simulink model "OkidniStepen"  (R2014b)
settings: Solver=ode5  StartTime=0.0  StopTime=0.1  FixedStep=10e-6  RelTol=1e-3
values from neighbouring files (symbols this model uses):
  f = 50    [Parametri.m]
  Vmax = 220*sqrt(2)    [Parametri.m]
settings Model: Creator=Zorana  LastModifiedBy=Zorana

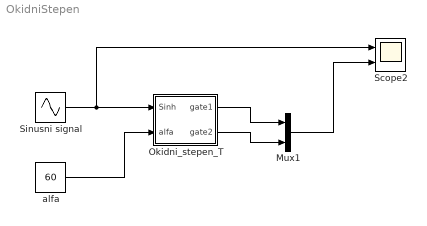
== system OkidniStepen ==
  Mux1 : Mux  Inputs=2
  Okidni_stepen_T : Subsystem
  Scope2 : Scope  NumInputPorts=2
      settings: YMin=-5~-5  YMax=15~5  SaveName=ScopeData2
  Sinusni signal : Sin  Amplitude=Vmax  Frequency=f*2*pi  SampleTime=0
  alfa : Constant  Value=60
  wires:
  Sinusni signal/1 -> Scope2/1, Okidni_stepen_T/1(Sinh)
  alfa/1 -> Okidni_stepen_T/2(alfa)
  Okidni_stepen_T/1(gate1) -> Mux1/1
  Okidni_stepen_T/2(gate2) -> Mux1/2
  Mux1/1 -> Scope2/2

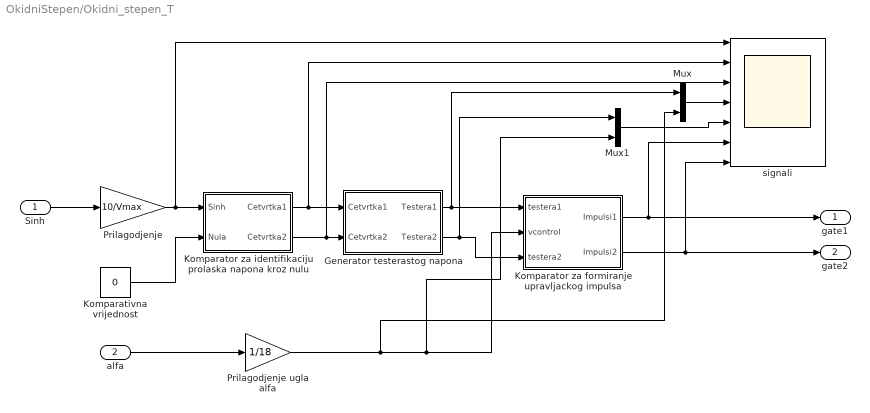
== system OkidniStepen/Okidni_stepen_T ==
  Sinh : Inport
  alfa : Inport  Port=2
  Generator testerastog napona : Subsystem
  Komparativna vrijednost : Constant  Value=0
  Komparator za formiranje upravljackog impulsa : Subsystem
  Komparator za identifikaciju prolaska napona kroz nulu : Subsystem
  Mux : Mux  Inputs=2
  Mux1 : Mux  Inputs=2
  Prilagodjenje : Gain  Gain=10/Vmax
  Prilagodjenje ugla alfa : Gain  Gain=1/18
  signali : Scope  NumInputPorts=7
      settings: YMin=-10~0~0~0~-5~0~0  YMax=10~11~11~11~5~11~11  SaveName=ScopeData3
  gate1 : Outport
  gate2 : Outport  Port=2
  wires:
  Komparator za formiranje upravljackog impulsa/1(Impulsi1) -> signali/6, gate1/1
  Komparator za identifikaciju prolaska napona kroz nulu/1(Cetvrtka1) -> signali/2, Generator testerastog napona/1(Cetvrtka1)
  Sinh/1 -> Prilagodjenje/1
  Prilagodjenje ugla alfa/1 -> Mux/2, Mux1/2, Komparator za formiranje upravljackog impulsa/2(vcontrol)
  Prilagodjenje/1 -> signali/1, Komparator za identifikaciju prolaska napona kroz nulu/1(Sinh)
  Generator testerastog napona/1(Testera1) -> Mux/1, Komparator za formiranje upravljackog impulsa/1(testera1)
  alfa/1 -> Prilagodjenje ugla alfa/1
  Komparativna vrijednost/1 -> Komparator za identifikaciju prolaska napona kroz nulu/2(Nula)
  Komparator za identifikaciju prolaska napona kroz nulu/2(Cetvrtka2) -> signali/3, Generator testerastog napona/2(Cetvrtka2)
  Generator testerastog napona/2(Testera2) -> Mux1/1, Komparator za formiranje upravljackog impulsa/3(testera2)
  Komparator za formiranje upravljackog impulsa/2(Impulsi2) -> signali/7, gate2/1
  Mux/1 -> signali/4
  Mux1/1 -> signali/5

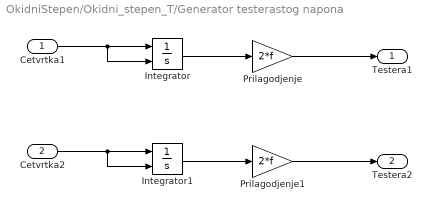
== system OkidniStepen/Okidni_stepen_T/Generator testerastog napona ==
  Cetvrtka1 : Inport
  Cetvrtka2 : Inport  Port=2
  Integrator : Integrator  ExternalReset=either
  Integrator1 : Integrator  ExternalReset=either
  Prilagodjenje : Gain  Gain=2*f
  Prilagodjenje1 : Gain  Gain=2*f
  Testera1 : Outport
  Testera2 : Outport  Port=2
  wires:
  Integrator/1 -> Prilagodjenje/1
  Cetvrtka1/1 -> Integrator/1, Integrator/2
  Prilagodjenje/1 -> Testera1/1
  Integrator1/1 -> Prilagodjenje1/1
  Cetvrtka2/1 -> Integrator1/2, Integrator1/1
  Prilagodjenje1/1 -> Testera2/1

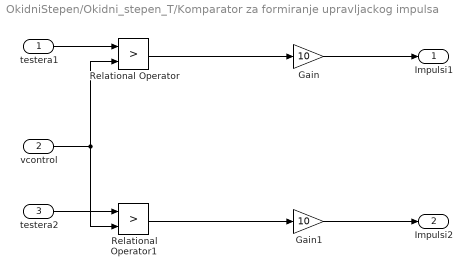
== system OkidniStepen/Okidni_stepen_T/Komparator za formiranje upravljackog impulsa ==
  testera1 : Inport
  vcontrol : Inport  Port=2
  testera2 : Inport  Port=3
  Gain : Gain  Gain=10
  Gain1 : Gain  Gain=10
  Relational Operator : RelationalOperator  Operator=>  OutDataTypeStr=fixdt(1,16)  InputSameDT=on
  Relational Operator1 : RelationalOperator  Operator=>  OutDataTypeStr=fixdt(1,16)  InputSameDT=on
  Impulsi1 : Outport
  Impulsi2 : Outport  Port=2
  wires:
  vcontrol/1 -> Relational Operator/2, Relational Operator1/2
  testera1/1 -> Relational Operator/1
  Gain/1 -> Impulsi1/1
  testera2/1 -> Relational Operator1/1
  Gain1/1 -> Impulsi2/1
  Relational Operator/1 -> Gain/1
  Relational Operator1/1 -> Gain1/1

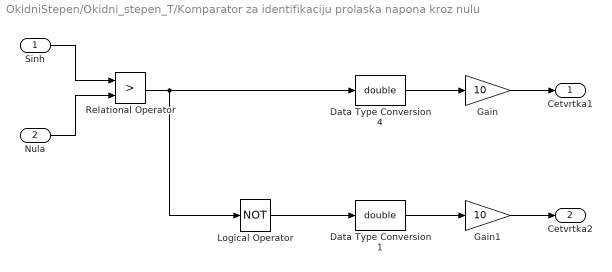
== system OkidniStepen/Okidni_stepen_T/Komparator za identifikaciju prolaska napona kroz nulu ==
  Sinh : Inport
  Nula : Inport  Port=2
  Data Type Conversion1 : DataTypeConversion  OutDataTypeStr=double  SaturateOnIntegerOverflow=on  RndMeth=Zero
  Data Type Conversion4 : DataTypeConversion  OutDataTypeStr=double  SaturateOnIntegerOverflow=on  RndMeth=Zero
  Gain : Gain  Gain=10
  Gain1 : Gain  Gain=10
  Logical Operator : Logic  Operator=NOT  IconShape=distinctive  AllPortsSameDT=off  OutDataTypeStr=boolean
  Relational Operator : RelationalOperator  Operator=>  OutDataTypeStr=fixdt(1,16)  InputSameDT=on
  Cetvrtka1 : Outport
  Cetvrtka2 : Outport  Port=2
  wires:
  Gain/1 -> Cetvrtka1/1
  Sinh/1 -> Relational Operator/1
  Nula/1 -> Relational Operator/2
  Relational Operator/1 -> Logical Operator/1, Data Type Conversion4/1
  Data Type Conversion4/1 -> Gain/1
  Gain1/1 -> Cetvrtka2/1
  Data Type Conversion1/1 -> Gain1/1
  Logical Operator/1 -> Data Type Conversion1/1
